simulink subsystem "neuralNetInference"  (R2021a)
settings: Solver=VariableStepAuto  StartTime=0.0  StopTime=10.0  RelTol=1e-3
values from neighbouring files (symbols this model uses):
  biasesLayer1 = model.LayerBiases{1}    [gatherNnetCodegenConstants.m]
  biasesLayer2 = model.LayerBiases{2}    [gatherNnetCodegenConstants.m]
  params = bestParams    [trainNet.m]
  trainingMean = mean(trainingFeatures, 1)    [computeInputNormalizationFactors.m]    (also in convertNetToONNX.m = varfun(@(f) mean(f, 'omitnan'), trainingFeatures, 'OutputFor)
  trainingStdInv = 1./trainingStd    [gatherNnetCodegenConstants.m]
  weightsLayer1 = model.LayerWeights{1}    [gatherNnetCodegenConstants.m]
  weightsLayer2 = model.LayerWeights{2}    [gatherNnetCodegenConstants.m]
settings Model: Creator=trevor  LastModifiedBy=trevor

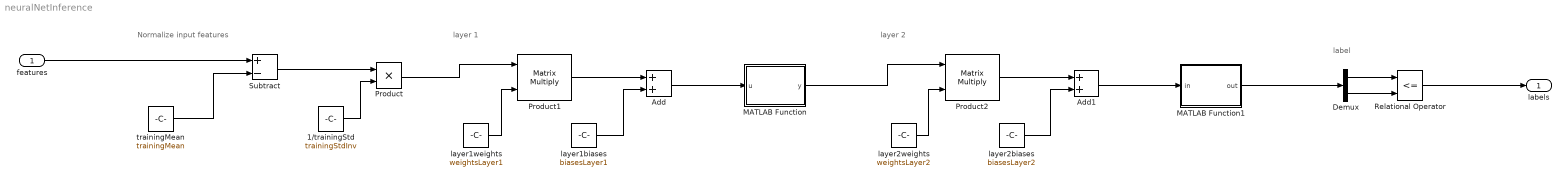
== system neuralNetInference ==
  note: label
  note: layer 1
  note: Normalize input features
  note: layer 2
  features : Inport
  1/trainingStd : Constant  Value=trainingStdInv  SampleTime=params.systemClockPeriod
  Add : Sum
  Add1 : Sum
  Demux : Demux  Outputs=2
  MATLAB Function : MATLAB Function  TreatAsAtomicUnit=on
  MATLAB Function1 : MATLAB Function  TreatAsAtomicUnit=on
  Product : Product
  Product1 : Product  Multiplication=Matrix(*)
  Product2 : Product  Multiplication=Matrix(*)
  Relational Operator : RelationalOperator  Operator=<=  OutDataTypeStr=boolean  RndMeth=Simplest
  Subtract : Sum  Inputs=+-
  layer1biases : Constant  Value=biasesLayer1  SampleTime=params.systemClockPeriod
  layer1weights : Constant  Value=weightsLayer1  SampleTime=params.systemClockPeriod
  layer2biases : Constant  Value=biasesLayer2  SampleTime=params.systemClockPeriod
  layer2weights : Constant  Value=weightsLayer2  SampleTime=params.systemClockPeriod
  trainingMean : Constant  Value=trainingMean  SampleTime=params.systemClockPeriod
  labels : Outport
  wires:
  Subtract/1 -> Product/1
  layer2weights/1 -> Product2/2
  Relational Operator/1 -> labels/1
  features/1 -> Subtract/1
  1/trainingStd/1 -> Product/2
  Demux/1 -> Relational Operator/1
  Add/1 -> MATLAB Function/1(u)
  MATLAB Function1/1(out) -> Demux/1
  Add1/1 -> MATLAB Function1/1(in)
  Product1/1 -> Add/1
  trainingMean/1 -> Subtract/2
  Product/1 -> Product1/1
  MATLAB Function/1(y) -> Product2/1
  layer1biases/1 -> Add/2
  Demux/2 -> Relational Operator/2
  Product2/1 -> Add1/1
  layer2biases/1 -> Add1/2
  layer1weights/1 -> Product1/2

== matlab function neuralNetInference/MATLAB Function ==
  data: u input; y output
function y = sigmoid(u)
%#codegen

y = 1./(1 + exp(-u));

== matlab function neuralNetInference/MATLAB Function1 ==
  data: in input; out output
function out  = softmax(in)
%#codgen

expIn = exp(in);

% TODO: it'd be nice to get rid of this division if possible
out = (expIn) / sum(expIn);

end
